simulink model "againGroundMPC"  (R2018a)
settings: Solver=ode1  StartTime=0.0  StopTime=10  FixedStep=Ts  RelTol=1e-3
values from neighbouring files (symbols this model uses):
  ground_W = diag([10 1 10 0.1 0.1])    [setupSimulink.m]
  ground_WN = diag([20 10 10])    [setupSimulink.m]
undefined symbols (not defined in the file or in its folder): ground_j0, groundParams, NR, object_ref, object_ref_rpy
settings Model: Creator=nicola  LastModifiedBy=nicola

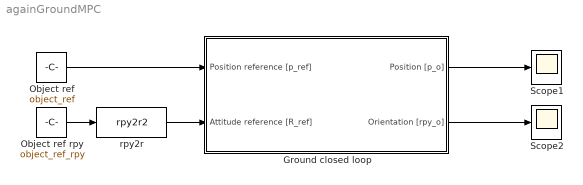
== system againGroundMPC ==
  Ground closed loop : Subsystem
  Object ref : Constant  Value=object_ref
  Object ref rpy : Constant  Value=object_ref_rpy
  Scope1 : Scope
  Scope2 : Scope
  rpy2r : MATLABFcn  MATLABFcn=rpy2r2  Output1D=off
  wires:
  Ground closed loop/1(Position [p_o]) -> Scope1/1
  Object ref/1 -> Ground closed loop/1(Position reference [p_ref])
  Object ref rpy/1 -> rpy2r/1
  rpy2r/1 -> Ground closed loop/2(Attitude reference [R_ref])
  Ground closed loop/2(Orientation [rpy_o]) -> Scope2/1

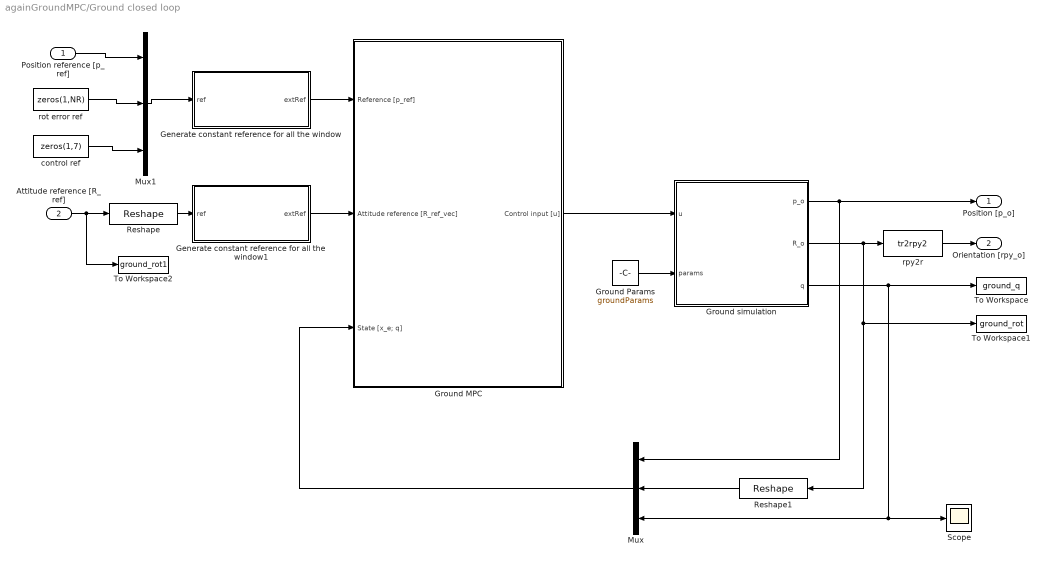
== system againGroundMPC/Ground closed loop ==
  Position reference [p_ref] : Inport
  Attitude reference [R_ref] : Inport  Port=2
  Generate constant reference for all the window : MATLAB Function  TreatAsAtomicUnit=on
  Generate constant reference for all the window1 : MATLAB Function  TreatAsAtomicUnit=on
  Ground MPC : Subsystem
  Ground Params : Constant  Value=groundParams
  Ground simulation : Subsystem
  Mux : Mux  Inputs=3
  Mux1 : Mux  Inputs=3
  Reshape : Reshape
  Reshape1 : Reshape
  Scope : Scope
  To Workspace : ToWorkspace  VariableName=ground_q  SaveFormat=Structure With Time  SampleTime=-1
  To Workspace1 : ToWorkspace  VariableName=ground_rot  SampleTime=-1
  To Workspace2 : ToWorkspace  VariableName=ground_rot1  SampleTime=-1
  control ref : Constant  Value=zeros(1,7)
  rot error ref : Constant  Value=zeros(1,NR)
  rpy2r : MATLABFcn  MATLABFcn=tr2rpy2
  Position [p_o] : Outport
  Orientation [rpy_o] : Outport  Port=2
  wires:
  Ground simulation/3(q) -> To Workspace/1, Scope/1, Mux/3
  Ground Params/1 -> Ground simulation/2(params)
  Generate constant reference for all the window/1(extRef) -> Ground MPC/1(Reference [p_ref])
  Position reference [p_ref]/1 -> Mux1/1
  Ground simulation/1(p_o) -> Mux/1, Position [p_o]/1
  Mux/1 -> Ground MPC/3(State [x_e; q])
  Ground MPC/1("Control input [u] ") -> Ground simulation/1(u)
  Mux1/1 -> Generate constant reference for all the window/1(ref)
  control ref/1 -> Mux1/3
  rot error ref/1 -> Mux1/2
  Attitude reference [R_ref]/1 -> To Workspace2/1, Reshape/1
  Reshape/1 -> Generate constant reference for all the window1/1(ref)
  Generate constant reference for all the window1/1(extRef) -> Ground MPC/2(Attitude reference [R_ref_vec])
  Ground simulation/2(R_o) -> rpy2r/1, To Workspace1/1, Reshape1/1
  Reshape1/1 -> Mux/2
  rpy2r/1 -> Orientation [rpy_o]/1

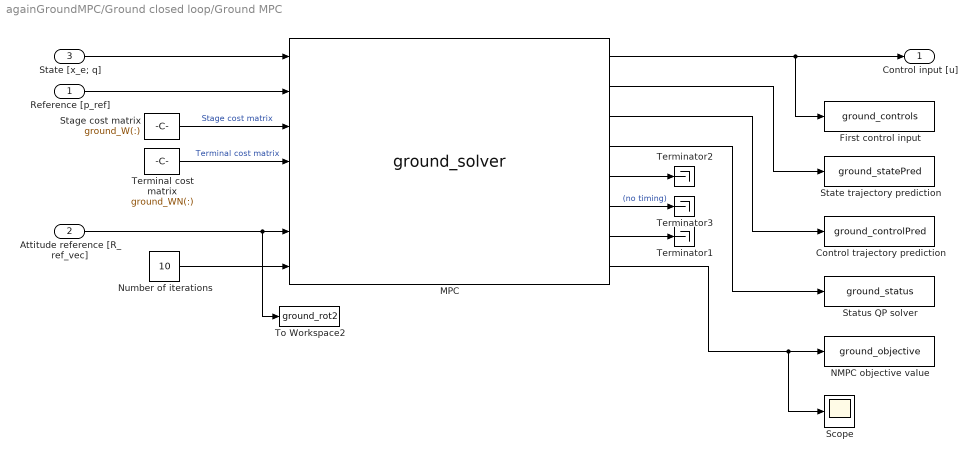
== system againGroundMPC/Ground closed loop/Ground MPC ==
  Reference [p_ref] : Inport
  Attitude reference [R_ref_vec] : Inport  Port=2
  State [x_e; q] : Inport  Port=3
  Control trajectory prediction : ToWorkspace  VariableName=ground_controlPred  SaveFormat=Structure With Time  SampleTime=-1
  First control input : ToWorkspace  VariableName=ground_controls  SaveFormat=Structure With Time  SampleTime=-1
  MPC : S-Function  FunctionName=ground_solver  Parameters=ground_xInit, ground_zInit, ground_uInit, ground_W, ground_WN, ground_bValues  SFunctionDeploymentMode=off  EnableBusSupport=off  mask(Legacy Function){SFunctionSpec=acado_step(ACADOinput u1[1], ACADOoutput y1[1]), ShowSpec=off}
      mask prompts: ShowSpec "Display function specification"
      mask help:
      | This block allows you to call the legacy functions specified by the following Legacy Code Tool definition:
      | def.SFunctionName = 'acado_solver_sfun';
      | def.OutputFcnSpec = 'acado_step(ACADOinput u1[1], ACADOoutput y1[1])';
      | def.StartFcnSpec = 'acado_initialize( void )';
      | def.TerminateFcnSpec = 'acado_cleanup( void )';
      | def.HeaderFiles = {'acado_common.h', 'acado_solver_sfunction.h'};
      | def.SourceFiles = {'acado_solver.c', 'acado_integrator.c', 'acado_auxiliary_functions.c', 'acado_solver_sfunction.c', 'acado_qpoases_interface.cpp', 'qpoases/SRC/Bounds.cpp', 'qpoases/SRC/Constraints.cpp', 'qpoases/SRC/CyclingManager.cpp', 'qpoases/SRC/Indexlist.cpp', 'qpoases/SRC/MessageHandling.cpp', 'qpoases/SRC/QProblem.cpp', 'qpoases/SRC/QProblemB.cpp', 'qpoases/SRC/SubjectTo.cpp', 'qpoases/SRC/Utils.cpp', 'qpoases/SRC/EXTRAS/SolutionAnalysis.cpp'};
      | def.IncPaths = {'qpoases', 'qpoases/INCLUDE', 'qpoases/SRC'};
      | def.Options.language = 'C++';
      mask Help: <p>This block was generated automatically by the Legacy Code Tool. For detailed help on this tool, call<a href="matlab:legacy_code('help')"> legacy_code('help')</a>.</p>
      mask Callback ShowSpec:
      | if strcmp(get_param(gcbh, 'ShowSpec'), 'on')
      |   set_param(gcbh, 'MaskDisplay', sprintf('fprintf(''%s'');', get_param(gcbh, 'SFunctionSpec')));
      | else
      |   set_param(gcbh, 'MaskDisplay', sprintf('fprintf(''%s'');', get_param(gcbh, 'FunctionName')));
      | end
      mask Display: fprintf('ground_solver');
  NMPC objective value : ToWorkspace  VariableName=ground_objective  SaveFormat=Structure With Time  SampleTime=-1
  Number of iterations : Constant  Value=10  OutDataTypeStr=double
  Scope : Scope
  Stage cost matrix : Constant  Value=ground_W(:)  OutDataTypeStr=double
  State trajectory prediction : ToWorkspace  VariableName=ground_statePred  SaveFormat=Structure With Time  SampleTime=-1
  Status QP solver : ToWorkspace  VariableName=ground_status  SaveFormat=Structure With Time  SampleTime=-1
  Terminal cost matrix : Constant  Value=ground_WN(:)  OutDataTypeStr=double
  Terminator1 : Terminator
  Terminator2 : Terminator
  Terminator3 : Terminator
  To Workspace2 : ToWorkspace  VariableName=ground_rot2  SampleTime=-1
  "Control input [u] " : Outport
  wires:
  MPC/3 -> Control trajectory prediction/1
  MPC/7 -> Terminator1/1
  Stage cost matrix/1 -> MPC/3  "Stage cost matrix"
  MPC/4 -> Status QP solver/1
  MPC/5 -> Terminator2/1
  MPC/1 -> "Control input [u] "/1, First control input/1
  Number of iterations/1 -> MPC/7
  MPC/8 -> Scope/1, NMPC objective value/1
  Terminal cost matrix/1 -> MPC/4  "Terminal cost matrix"
  MPC/2 -> State trajectory prediction/1
  MPC/6 -> Terminator3/1  "(no timing)"
  State [x_e; q]/1 -> MPC/1
  Reference [p_ref]/1 -> MPC/2
  Attitude reference [R_ref_vec]/1 -> To Workspace2/1, MPC/6

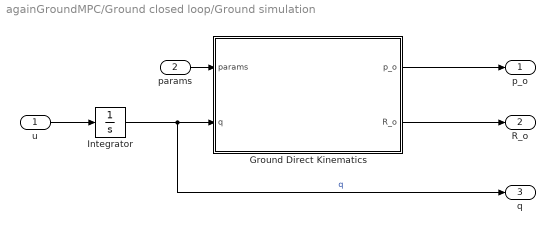
== system againGroundMPC/Ground closed loop/Ground simulation ==
  u : Inport
  params : Inport  Port=2
  Ground Direct Kinematics : MATLAB Function  TreatAsAtomicUnit=on
  Integrator : Integrator  InitialCondition=ground_j0
  p_o : Outport
  R_o : Outport  Port=2
  q : Outport  Port=3
  wires:
  params/1 -> Ground Direct Kinematics/1(params)
  Integrator/1 -> Ground Direct Kinematics/2(q), q/1  "q"
  Ground Direct Kinematics/1(p_o) -> p_o/1
  u/1 -> Integrator/1
  Ground Direct Kinematics/2(R_o) -> R_o/1

== matlab function againGroundMPC/Ground closed loop/Ground simulation/Ground Direct Kinematics ==
  data: params input; p_o output size=3; q input size=7; R_o output size=3,3
function [p_o, R_o] = groundKinematics (params, q)
    T = T_w_o (params, q);
    [R_o, p_o] = tr2rt (T);
end

function T = T_w_o (params, q)
   T = reshape([cos(q(2)+q(3)+q(4)).*cos(q(7)+q(1)),cos(q(2)+q(3)+q(4)).*sin(q(7)+q(1)),sin(q(2)+q(3)+q(4)),0.0,-sin(q(2)+q(3)+q(4)).*cos(q(7)+q(1)),-sin(q(2)+q(3)+q(4)).*sin(q(7)+q(1)),cos(q(2)+q(3)+q(4)),0.0,sin(q(7)+q(1)),-cos(q(7)+q(1)),0.0,0.0,q(5)+params(4).*(cos(q(7)+q(1)).*cos(q(2)+q(3)).*cos(q(4))-cos(q(7)+q(1)).*sin(q(2)+q(3)).*sin(q(4)))-params(5).*(cos(q(7)+q(1)).*cos(q(2)+q(3)).*sin(q(4))+cos(q(7)+q(1)).*sin(q(2)+q(3)).*cos(q(4)))+params(6).*sin(q(7)+q(1))+params(2).*cos(q(7)+q(1)).*cos(q(2)+q(3))+params(1).*cos(q(7)+q(1)).*cos(q(2))-params(3).*cos(q(7)+q(1)).*sin(q(2)+q(3)).*sin(q(4))+params(3).*cos(q(7)+q(1)).*cos(q(2)+q(3)).*cos(q(4)),q(6)-params(6).*cos(q(7)+q(1))+params(4).*(cos(q(2)+q(3)).*sin(q(7)+q(1)).*cos(q(4))-sin(q(7)+q(1)).*sin(q(2)+q(3)).*sin(q(4)))-params(5).*(cos(q(2)+q(3)).*sin(q(7)+q(1)).*sin(q(4))+sin(q(7)+q(1)).*sin(q(2)+q(3)).*cos(q(4)))+params(2).*cos(q(2)+q(3)).*sin(q(7)+q(1))+params(1).*sin(q(7)+q(1)).*cos(q(2))+params(3).*cos(q(2)+q(3)).*sin(q(7)+q(1)).*cos(q(4))-params(3).*sin(q(7)+q(1)).*sin(q(2)+q(3)).*sin(q(4)),params(2).*sin(q(2)+q(3))+params(1).*sin(q(2))+params(5).*cos(q(2)+q(3)+q(4))+params(3).*sin(q(2)+q(3)+q(4))+params(4).*sin(q(2)+q(3)+q(4)),1.0],[4,4]);
end

== matlab function againGroundMPC/Ground closed loop/Generate constant reference for all the window ==
  data: ref input double; extRef output
function extRef = constReference (ref)
    % Need to be hardcoded each time
    N = 10;
    
    ref = reshape (ref,length(ref),1);
    yN = ref(1:end-7);
    y = [repmat(ref',N,1)].';
    extRef = [y(:);yN];
end

== matlab function againGroundMPC/Ground closed loop/Generate constant reference for all the window1 ==
  data: ref input double; extRef output
function extRef = constReference (ref)
    % Need to be hardcoded each time
    N = 10;
    
    ref = reshape (ref,length(ref),1);
    yN = ref;
    y = [repmat(ref',N+1,1)].';
    extRef = [y(:)];
end
